simulink model "measure_delay"  (R2023b)
settings: Solver=FixedStepDiscrete  StartTime=0.0  StopTime=200  RelTol=1e-3
libraries: simulink x4, hdlsllib x3
settings Model: DataTypeOverride=Off  Creator=tcollins  LastModifiedBy=tcollins
settings SolverCC: AlgebraicLoopSolver=TrustRegion
settings DataIOCC: LimitDataPoints=on  SaveOutput=off  SaveTime=off
settings OptimizationCC: BlockReduction=off  ConditionallyExecuteInputs=off  DefaultParameterBehavior=Inlined  LifeSpan=inf
settings DebuggingCC: AlgebraicLoopMsg=error  SingleTaskRateTransMsg=error  UnconnectedInputMsg=warning  UnconnectedOutputMsg=warning  UnconnectedLineMsg=warning  AllowSymbolicDim=off  StrictBusMsg=ErrorOnBusTreatedAsVector  SFUnexpectedBacktrackingDiag=warning  SFNoUnconditionalDefaultTransitionDiag=warning  SFExecutionAtInitializationDiag=none  ArithmeticOperatorsInVariantConditions=warning
settings HardwareCC: ProdBitPerPointer=32  ProdBitPerSizeT=32  ProdBitPerPtrDiffT=32  ProdLargestAtomicFloat=None  ProdIntDivRoundTo=Undefined  ProdEndianess=Unspecified  ProdWordSize=32  ProdHWDeviceType=ASIC/FPGA->ASIC/FPGA  ProdEqTarget=off
settings ModelReferenceCC: EnableRefExpFcnMdlSchedulingChecks=on
settings SFSimCC: SimUseLocalCustomCode=off  CustomCodeUndefinedFunction=UseInterfaceOnly
settings RTWCC: RTWUseLocalCustomCode=off
settings CodeAppCC: StateflowObjectComments=on
settings GRTTargetCC: TargetLangStandard=C89/C90 (ANSI)
settings ConfigComp: CovScope=ReferencedModels  CovMetricSettings=dw  CovSaveCumulativeToWorkspaceVar=on  CovSaveSingleToWorkspaceVar=on  CovExternalEMLEnable=off  CovSFcnEnable=off

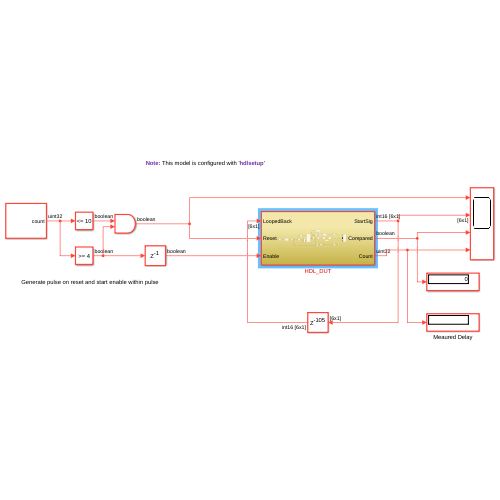
[thumbnail: Simulink's stored preview of the top-level diagram]
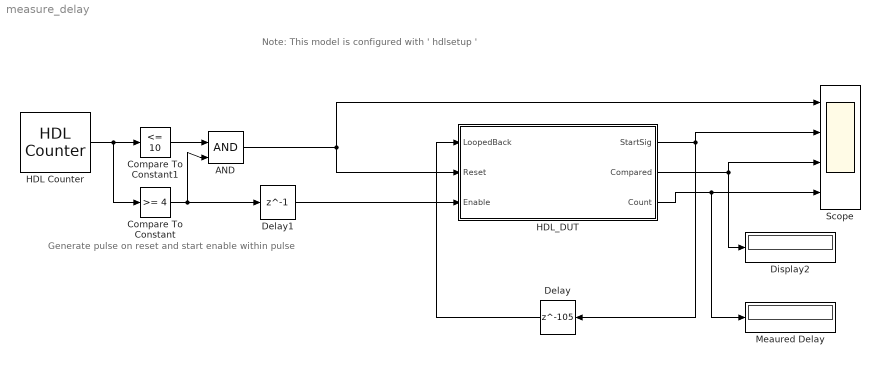
== system measure_delay ==
  note: Generate pulse on reset and start enable within pulse
  note: Note: This model is configured with ' hdlsetup '
  AND : Logic  IconShape=distinctive  AllPortsSameDT=off  OutDataTypeStr=boolean
  Compare To Constant : simulink/Logic and Bit Operations/Compare To Constant  relop=>=  const=4  OutDataTypeStr=boolean
  Compare To Constant1 : simulink/Logic and Bit Operations/Compare To Constant  relop=<=  const=10  OutDataTypeStr=boolean
  Delay : Delay  DelayLength=105
  Delay1 : Delay  DelayLength=1
  Display2 : Display
  HDL Counter : hdlsllib/Sources/HDL Counter  CountType=Count limited  CountInit=0  CountStep=1  CountMax=10000  CountFromType=Initial value  CountFrom=0  CountResetPort=off  CountLoadPort=off  CountEnbPort=off  CountDirPort=off  CountHitOutputPort=off  CountDataType=Unsigned  CountWordLen=32  CountFracLen=0  CountSampTime=1
  HDL_DUT : Subsystem
  Meaured Delay : Display
  Scope : Scope  NumInputPorts=4
  wires:
  HDL_DUT/1(StartSig) -> Delay/1, Scope/2
  Delay/1 -> HDL_DUT/1(LoopedBack)
  HDL_DUT/2(Compared) -> Display2/1, Scope/3
  HDL Counter/1 -> Compare To Constant/1, Compare To Constant1/1
  Compare To Constant/1 -> Delay1/1, AND/2
  HDL_DUT/3(Count) -> Meaured Delay/1, Scope/4
  AND/1 -> HDL_DUT/2(Reset), Scope/1
  Delay1/1 -> HDL_DUT/3(Enable)
  Compare To Constant1/1 -> AND/1

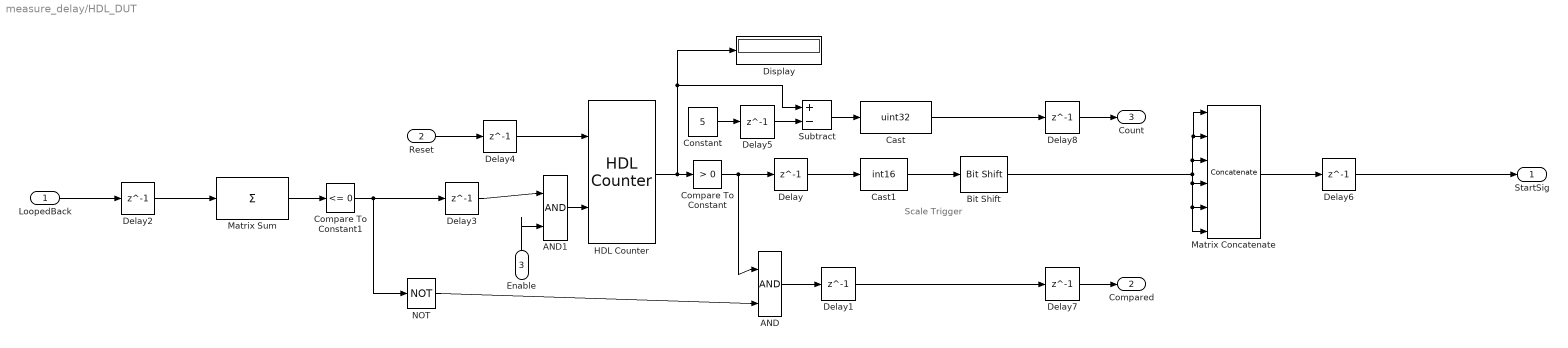
== system measure_delay/HDL_DUT ==
  note: Scale Trigger
  LoopedBack : Inport
  Reset : Inport  Port=2
  Enable : Inport  Port=3
  AND : Logic  IconShape=distinctive  AllPortsSameDT=off  OutDataTypeStr=boolean
  AND1 : Logic  IconShape=distinctive  AllPortsSameDT=off  OutDataTypeStr=boolean
  Bit Shift : hdlsllib/Logic and Bit Operations/Bit Shift  mode=Shift Left Logical  N=6
  Cast : DataTypeConversion  OutDataTypeStr=uint32  ConvertRealWorld=Stored Integer (SI)  RndMeth=Floor
  Cast1 : DataTypeConversion  OutDataTypeStr=int16  ConvertRealWorld=Stored Integer (SI)  RndMeth=Floor
  Compare To Constant : simulink/Logic and Bit Operations/Compare To Constant  relop=>  const=0  OutDataTypeStr=boolean
  Compare To Constant1 : simulink/Logic and Bit Operations/Compare To Constant  relop=<=  const=0  OutDataTypeStr=boolean
  Constant : Constant  Value=5  OutDataTypeStr=uint8  SampleTime=-1
  Delay{,1..8} (9 alike) : Delay  DelayLength=1
  Display : Display
  HDL Counter : hdlsllib/Sources/HDL Counter  CountType=Count limited  CountInit=0  CountStep=1  CountMax=2^31  CountFromType=Initial value  CountFrom=0  CountResetPort=on  CountLoadPort=off  CountEnbPort=on  CountDirPort=off  CountHitOutputPort=off  CountDataType=Unsigned  CountWordLen=32  CountFracLen=0  CountSampTime=1
  Matrix Concatenate : Concatenate  NumInputs=6  Mode=Multidimensional array
  Matrix Sum : Sum  Inputs=+
  NOT : Logic  Operator=NOT  IconShape=distinctive  AllPortsSameDT=off  OutDataTypeStr=boolean
  Subtract : Sum  Inputs=+-
  StartSig : Outport  VectorParamsAs1DForOutWhenUnconnected=off
  Compared : Outport  Port=2  VectorParamsAs1DForOutWhenUnconnected=off
  Count : Outport  Port=3  VectorParamsAs1DForOutWhenUnconnected=off
  wires:
  Delay/1 -> Cast1/1
  Delay1/1 -> Delay7/1
  Compare To Constant/1 -> AND/1, Delay/1
  LoopedBack/1 -> Delay2/1
  Delay2/1 -> Matrix Sum/1
  AND/1 -> Delay1/1
  Reset/1 -> Delay4/1
  Delay4/1 -> HDL Counter/1
  Delay3/1 -> AND1/1
  AND1/1 -> HDL Counter/2
  Enable/1 -> AND1/2
  HDL Counter/1 -> Subtract/1, Display/1, Compare To Constant/1
  Compare To Constant1/1 -> Delay3/1, NOT/1
  NOT/1 -> AND/2
  Subtract/1 -> Cast/1
  Constant/1 -> Delay5/1
  Cast/1 -> Delay8/1
  Delay5/1 -> Subtract/2
  Bit Shift/1 -> Matrix Concatenate/2, Matrix Concatenate/1, Matrix Concatenate/3, Matrix Concatenate/6, Matrix Concatenate/5, Matrix Concatenate/4
  Cast1/1 -> Bit Shift/1
  Delay6/1 -> StartSig/1
  Delay7/1 -> Compared/1
  Delay8/1 -> Count/1
  Matrix Concatenate/1 -> Delay6/1
  Matrix Sum/1 -> Compare To Constant1/1
